simulink model "Task6"  (R2023b)
settings: Solver=FixedStepAuto  StartTime=0.0  StopTime=150  FixedStep=.02  RelTol=1e-3
InitFcn:
  | run("Linear_Model.m")
undefined symbols (not defined in the file or in its folder): A_Lat, A_Long, B_Lat, B_Long, C_Lat, C_Long, D_Lat, D_Long, gravity, sigbuilder_block, states_0, theta0, u0, w0
libraries: simulink_extras x42, cstblocks x27, slpidlib x8
(part 2 of 2)

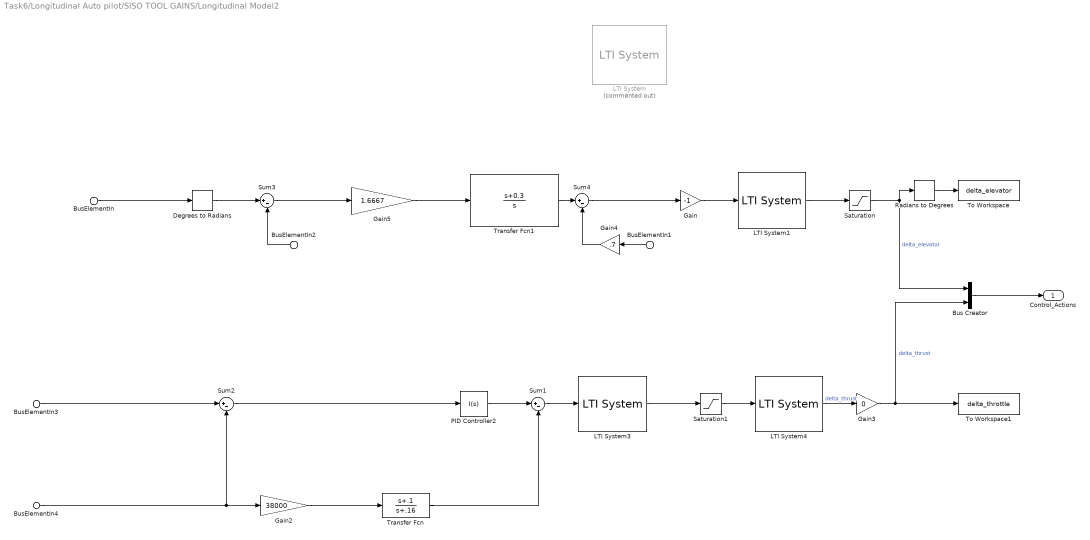
== system Task6/Longitudinal Auto pilot/SISO TOOL GAINS/Longitudinal Model2 ==
  BusElementIn1 : Inport  PortName=deltas  Element=deltas.delta_q
  BusElementIn2 : Inport  PortName=deltas  Element=deltas.delta_theta
  BusElementIn4 : Inport  PortName=deltas  Element=deltas.delta_u
  BusElementIn : Inport  Port=2  PortName=Commands  Element=commands.theta_command
  BusElementIn3 : Inport  Port=2  PortName=Commands  Element=commands.u_command
  Bus Creator : BusCreator  Inputs=2
  Degrees to Radians : simulink_extras/Transformations/Degrees to Radians
  Gain : Gain  Gain=-1
  Gain2 : Gain  Gain=38000
  Gain3 : Gain  Gain=0
  Gain4 : Gain  Gain=.7
  Gain5 : Gain  Gain=1.6667
  LTI System : cstblocks/LTI System  Commented=on  sys=PI_Pitch  IC=[]  PadeOrder=0
  LTI System1 : cstblocks/LTI System  sys=servo  IC=[]  PadeOrder=0
  LTI System3 : cstblocks/LTI System  sys=servo  IC=[]  PadeOrder=0
  LTI System4 : cstblocks/LTI System  sys=Engine_Lag  IC=[]  PadeOrder=0
  PID Controller2 : slpidlib/PID Controller  Controller=I  Form=Parallel  TimeDomain=Continuous-time  UseExternalTs=off  SampleTime=-1  IntegratorMethod=Forward Euler  FilterMethod=Forward Euler  ControllerParametersSource=internal  P=25000  I=1400  UseKiTs=off  D=45918.9077381397  N=24.6739321802593  UseFilter=on  TunerSelectOption=Transfer Function Based (PID Tuner App)  InitialConditionSource=internal  InitialConditionForIntegrator=0  InitialConditionForFilter=0  DifferentiatorICPrevScaledInput=0  ExternalReset=none  TrackingMode=off  Kt=1  LimitOutput=off  SatLimitsSource=internal  UpperSaturationLimit=inf  LowerSaturationLimit=-inf  LinearizeAsGain=on  AntiWindupMode=none  Kb=1  LimitIntegrator=off  UpperIntegratorSaturationLimit=inf  LowerIntegratorSaturationLimit=-inf  POutMin=[]  POutMax=[]  IOutMin=[]  IOutMax=[]  DOutMin=[]  DOutMax=[]  NOutMin=[]  NOutMax=[]  SumOutMin=[]  SumOutMax=[]  SaturationOutMin=[]  SaturationOutMax=[]  PParamMin=[]  PParamMax=[]  IParamMin=[]  IParamMax=[]  DParamMin=[]  DParamMax=[]  NParamMin=[]  NParamMax=[]  KbParamMin=[]  KbParamMax=[]  KtParamMin=[]  KtParamMax=[]  KbOutMin=[]  KbOutMax=[]  KtOutMin=[]  KtOutMax=[]  IntegratorOutMin=[]  IntegratorOutMax=[]  FilterOutMin=[]  FilterOutMax=[]  SumI1OutMin=[]  SumI1OutMax=[]  SumI2OutMin=[]  SumI2OutMax=[]  SumI3OutMin=[]  SumI3OutMax=[]  SumI4OutMin=[]  SumI4OutMax=[]  SumDOutMin=[]  SumDOutMax=[]  DifferentiatorOutMin=[]  DifferentiatorOutMax=[]  FilterDiffOutCoefMin=[]  FilterDiffOutCoefMax=[]  ReciprocalOutMin=[]  ReciprocalOutMax=[]  SumDenOutMin=[]  SumDenOutMax=[]  SumNumOutMin=[]  SumNumOutMax=[]  DivideOutMin=[]  DivideOutMax=[]  UdiffTsProdOutMin=[]  UdiffTsProdOutMax=[]  NTsProdOutMin=[]  NTsProdOutMax=[]  UintegralTsProdOutMin=[]  UintegralTsProdOutMax=[]  UngainTsProdOutMin=[]  UngainTsProdOutMax=[]  ClampingZeroOutDataTypeStr=Inherit: Inherit via back propagation  ClampingZeroOutMin=[]  ClampingZeroOutMax=[]  FilterDenConstantOutDataTypeStr=Inherit: Inherit via back propagation  FilterDenConstantOutMin=[]  FilterDenConstantOutMax=[]  PCopyOutDataTypeStr=Inherit: Inherit via back propagation  PCopyOutMin=[]  PCopyOutMax=[]  NCopyOutDataTypeStr=Inherit: Inherit via back propagation  NCopyOutMin=[]  NCopyOutMax=[]  IntegratorContinuousStateAttributes=''  IntegratorStateMustResolveToSignalObject=off  IntegratorRTWStateStorageClass=Auto  FilterContinuousStateAttributes=''  FilterStateMustResolveToSignalObject=off  FilterRTWStateStorageClass=Auto  ParallelPVariant=Disabled  IdealPVariant=Disabled  IVariant=InternalParameters  DVariant=Disabled  IntegratorVariant=Continuous  SatVariant=Disabled  AWVariant=Passthrough  PCopyVariant=Disabled  TRVariant=Disabled  FdbkBlocksVariant=Forward  IdealPFdbkVariant=Disabled  SatFdbkVariant=Disabled  DerivativeFilterVariant=Disabled  NVariant=Disabled  NCopyVariant=Disabled_SignalSpec  FilterICVariant=Disabled  IntegratorICVariant=InternalICs  ExternalResetVariant=Disabled  TRSumVariant=Passthrough  SumFdbkVariant=Disabled  SumVariant=Passthrough_I  TsampFilterVariant=InternalTs  TsampNgainVariant=Passthrough  TsampIntegralVariant=Disabled_SignalSpec  ExternalSaturationOutDataTypeStr=Inherit: Same as second input
  Radians to Degrees : simulink_extras/Transformations/Radians to Degrees
  Saturation : Saturate  UpperLimit=deg2rad(25)  LowerLimit=deg2rad(-25)
  Saturation1 : Saturate  UpperLimit=65369  LowerLimit=-269369.84
  Sum{1..4} (4 alike) : Sum  Inputs=|+-
  To Workspace : ToWorkspace  VariableName=delta_elevator  SampleTime=-1
  To Workspace1 : ToWorkspace  VariableName=delta_throttle  SampleTime=-1
  Transfer Fcn : TransferFcn  Numerator=[1 .1]  Denominator=[1 .16]
  Transfer Fcn1 : TransferFcn  Numerator=[1 0.3]  Denominator=[1 0]
  Control_Actions : Outport
  wires:
  BusElementIn/1 -> Degrees to Radians/1
  Degrees to Radians/1 -> Sum3/1
  Sum3/1 -> Gain5/1
  Gain/1 -> LTI System1/1
  LTI System1/1 -> Saturation/1
  Saturation/1 -> Bus Creator/1, Radians to Degrees/1  "delta_elevator"
  Bus Creator/1 -> Control_Actions/1
  Radians to Degrees/1 -> To Workspace/1
  Sum2/1 -> PID Controller2/1
  Sum1/1 -> LTI System3/1
  LTI System3/1 -> Saturation1/1
  Saturation1/1 -> LTI System4/1
  Transfer Fcn/1 -> Sum1/2
  LTI System4/1 -> Gain3/1  "delta_thrust"
  Gain2/1 -> Transfer Fcn/1
  PID Controller2/1 -> Sum1/1
  Gain3/1 -> Bus Creator/2, To Workspace1/1  "delta_thrust"
  BusElementIn2/1 -> Sum3/2
  BusElementIn1/1 -> Gain4/1
  BusElementIn3/1 -> Sum2/1
  BusElementIn4/1 -> Sum2/2, Gain2/1
  Gain4/1 -> Sum4/2
  Gain5/1 -> Transfer Fcn1/1
  Sum4/1 -> Gain/1
  Transfer Fcn1/1 -> Sum4/1

== system Task6/Longitudinal Auto pilot/SISO TOOL GAINS/State Space Model3 ==
  Control_Actions : Inport
  Bus Creator1 : BusCreator  Inputs=4
  Bus Selector : BusSelector  OutputSignals=delta_elevator,delta_thrust
  Demux : Demux
  Gain : Gain  Gain=0
  Manual Switch : ManualSwitch
  Mux : Mux  Inputs=2
  State-Space : StateSpace  A=A_Long  B=B_Long  C=C_Long  D=D_Long  InitialCondition=0
  Out Bus Element : Outport  PortName=deltas  Element=deltas
  wires:
  Demux/3 -> Bus Creator1/3  "delta_q"
  Mux/1 -> State-Space/1
  Demux/2 -> Bus Creator1/2  "delta_w"
  Demux/1 -> Bus Creator1/1  "delta_u"
  Bus Creator1/1 -> Out Bus Element/1
  State-Space/1 -> Demux/1
  Demux/4 -> Bus Creator1/4  "delta_theta"
  Manual Switch/1 -> Mux/2
  Gain/1 -> Manual Switch/2
  Control_Actions/1 -> Bus Selector/1
  Bus Selector/1 -> Mux/1  "<delta_elevator>"
  Bus Selector/2 -> Gain/1, Manual Switch/1  "<delta_thrust>"

== system Task6/Longitudinal Auto pilot/SISO TOOL GAINS/Subsystem ==
  Bus Creator2 : BusCreator  Inputs=2
  Constant4 : Constant  Value=15
  Constant5 : Constant  Value=10
  Out Bus Element : Outport  PortName=Commands  Element=commands
  wires:
  Constant4/1 -> Bus Creator2/1  "theta_command"
  Constant5/1 -> Bus Creator2/2  "u_command"
  Bus Creator2/1 -> Out Bus Element/1

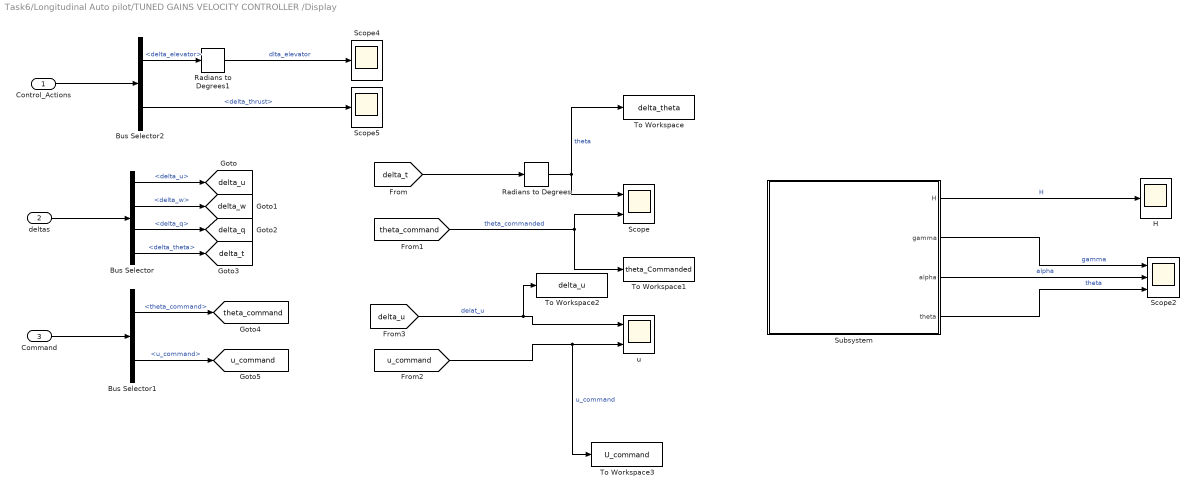
== system Task6/Longitudinal Auto pilot/TUNED GAINS VELOCITY CONTROLLER /Display ==
  Control_Actions : Inport
  deltas : Inport  Port=2
  Command : Inport  Port=3
  Bus Selector : BusSelector  OutputSignals=delta_u,delta_w,delta_q,delta_theta
  Bus Selector1 : BusSelector  OutputSignals=theta_command,u_command
  Bus Selector2 : BusSelector  OutputSignals=delta_elevator,delta_thrust
  H : Scope
  Radians to Degrees : simulink_extras/Transformations/Radians to Degrees
  Radians to Degrees1 : simulink_extras/Transformations/Radians to Degrees
  Scope : Scope  NumInputPorts=2
  Scope2 : Scope  NumInputPorts=3
  Scope4 : Scope
  Scope5 : Scope
  Subsystem : Subsystem
  To Workspace : ToWorkspace  VariableName=delta_theta  SampleTime=-1
  To Workspace1 : ToWorkspace  VariableName=theta_Commanded  SampleTime=-1
  To Workspace2 : ToWorkspace  VariableName=delta_u  SampleTime=-1
  To Workspace3 : ToWorkspace  VariableName=U_command  SampleTime=-1
  u : Scope  NumInputPorts=2
  tag scope: delta_q=global, delta_t=global, delta_u=global, delta_w=global, theta_command=global, u_command=global
  wires:
  deltas/1 -> Bus Selector/1
  Bus Selector/1 -> [delta_u]  "<delta_u>"
  Bus Selector/2 -> [delta_w]  "<delta_w>"
  Bus Selector/3 -> [delta_q]  "<delta_q>"
  Bus Selector/4 -> [delta_t]  "<delta_theta>"
  [delta_t] -> Radians to Degrees/1
  Radians to Degrees/1 -> To Workspace/1, Scope/1  "theta"
  [theta_command] -> To Workspace1/1, Scope/2  "theta_commanded"
  Subsystem/1(H) -> H/1  "H"
  Subsystem/3(alpha) -> Scope2/2  "alpha"
  Subsystem/2(gamma) -> Scope2/1  "gamma"
  Subsystem/4(theta) -> Scope2/3  "theta"
  Command/1 -> Bus Selector1/1
  Bus Selector1/1 -> [theta_command]  "<theta_command>"
  Bus Selector1/2 -> [u_command]  "<u_command>"
  [u_command] -> To Workspace3/1, u/2  "u_command"
  [delta_u] -> To Workspace2/1, u/1  "delat_u"
  Control_Actions/1 -> Bus Selector2/1
  Bus Selector2/1 -> Radians to Degrees1/1  "<delta_elevator>"
  Bus Selector2/2 -> Scope5/1  "<delta_thrust>"
  Radians to Degrees1/1 -> Scope4/1  "dlta_elevator"

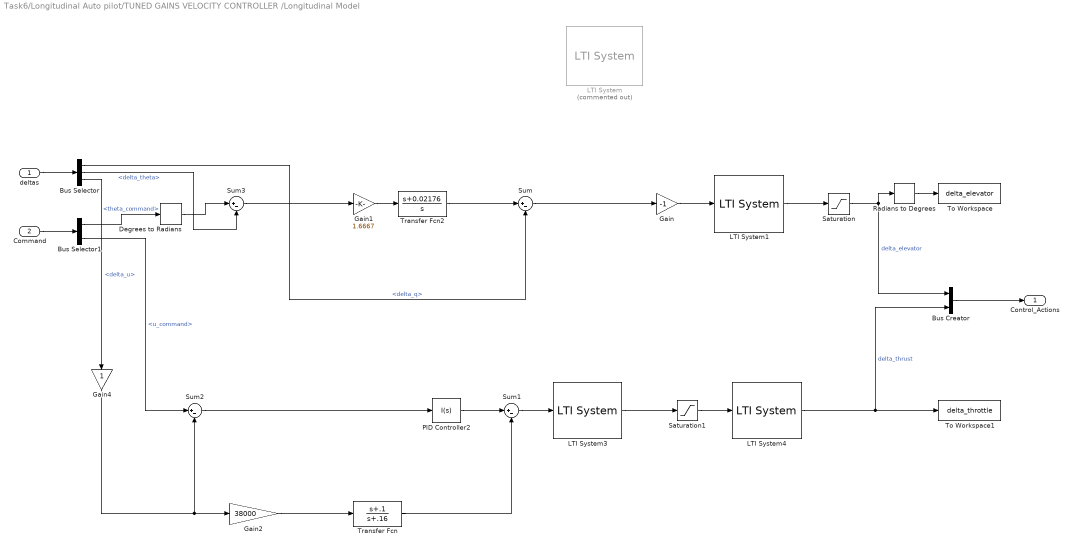
== system Task6/Longitudinal Auto pilot/TUNED GAINS VELOCITY CONTROLLER /Longitudinal Model ==
  deltas : Inport
  Command : Inport  Port=2
  Bus Creator : BusCreator  Inputs=2
  Bus Selector : BusSelector  OutputSignals=delta_q,delta_theta,delta_u
  Bus Selector1 : BusSelector  OutputSignals=theta_command,u_command
  Degrees to Radians : simulink_extras/Transformations/Degrees to Radians
  Gain : Gain  Gain=-1
  Gain1 : Gain  Gain=1.6667
  Gain2 : Gain  Gain=38000
  Gain4 : Gain
  LTI System : cstblocks/LTI System  Commented=on  sys=PI_Pitch  IC=[]  PadeOrder=0
  LTI System1 : cstblocks/LTI System  sys=servo  IC=[]  PadeOrder=0
  LTI System3 : cstblocks/LTI System  sys=servo  IC=[]  PadeOrder=0
  LTI System4 : cstblocks/LTI System  sys=Engine_Lag  IC=[]  PadeOrder=0
  PID Controller2 : slpidlib/PID Controller  Controller=I  Form=Parallel  TimeDomain=Continuous-time  UseExternalTs=off  SampleTime=-1  IntegratorMethod=Forward Euler  FilterMethod=Forward Euler  ControllerParametersSource=internal  P=25000  I=1400  UseKiTs=off  D=45918.9077381397  N=24.6739321802593  UseFilter=on  TunerSelectOption=Transfer Function Based (PID Tuner App)  InitialConditionSource=internal  InitialConditionForIntegrator=0  InitialConditionForFilter=0  DifferentiatorICPrevScaledInput=0  ExternalReset=none  TrackingMode=off  Kt=1  LimitOutput=off  SatLimitsSource=internal  UpperSaturationLimit=inf  LowerSaturationLimit=-inf  LinearizeAsGain=on  AntiWindupMode=none  Kb=1  LimitIntegrator=off  UpperIntegratorSaturationLimit=inf  LowerIntegratorSaturationLimit=-inf  POutMin=[]  POutMax=[]  IOutMin=[]  IOutMax=[]  DOutMin=[]  DOutMax=[]  NOutMin=[]  NOutMax=[]  SumOutMin=[]  SumOutMax=[]  SaturationOutMin=[]  SaturationOutMax=[]  PParamMin=[]  PParamMax=[]  IParamMin=[]  IParamMax=[]  DParamMin=[]  DParamMax=[]  NParamMin=[]  NParamMax=[]  KbParamMin=[]  KbParamMax=[]  KtParamMin=[]  KtParamMax=[]  KbOutMin=[]  KbOutMax=[]  KtOutMin=[]  KtOutMax=[]  IntegratorOutMin=[]  IntegratorOutMax=[]  FilterOutMin=[]  FilterOutMax=[]  SumI1OutMin=[]  SumI1OutMax=[]  SumI2OutMin=[]  SumI2OutMax=[]  SumI3OutMin=[]  SumI3OutMax=[]  SumI4OutMin=[]  SumI4OutMax=[]  SumDOutMin=[]  SumDOutMax=[]  DifferentiatorOutMin=[]  DifferentiatorOutMax=[]  FilterDiffOutCoefMin=[]  FilterDiffOutCoefMax=[]  ReciprocalOutMin=[]  ReciprocalOutMax=[]  SumDenOutMin=[]  SumDenOutMax=[]  SumNumOutMin=[]  SumNumOutMax=[]  DivideOutMin=[]  DivideOutMax=[]  UdiffTsProdOutMin=[]  UdiffTsProdOutMax=[]  NTsProdOutMin=[]  NTsProdOutMax=[]  UintegralTsProdOutMin=[]  UintegralTsProdOutMax=[]  UngainTsProdOutMin=[]  UngainTsProdOutMax=[]  ClampingZeroOutDataTypeStr=Inherit: Inherit via back propagation  ClampingZeroOutMin=[]  ClampingZeroOutMax=[]  FilterDenConstantOutDataTypeStr=Inherit: Inherit via back propagation  FilterDenConstantOutMin=[]  FilterDenConstantOutMax=[]  PCopyOutDataTypeStr=Inherit: Inherit via back propagation  PCopyOutMin=[]  PCopyOutMax=[]  NCopyOutDataTypeStr=Inherit: Inherit via back propagation  NCopyOutMin=[]  NCopyOutMax=[]  IntegratorContinuousStateAttributes=''  IntegratorStateMustResolveToSignalObject=off  IntegratorRTWStateStorageClass=Auto  FilterContinuousStateAttributes=''  FilterStateMustResolveToSignalObject=off  FilterRTWStateStorageClass=Auto  ParallelPVariant=Disabled  IdealPVariant=Disabled  IVariant=InternalParameters  DVariant=Disabled  IntegratorVariant=Continuous  SatVariant=Disabled  AWVariant=Passthrough  PCopyVariant=Disabled  TRVariant=Disabled  FdbkBlocksVariant=Forward  IdealPFdbkVariant=Disabled  SatFdbkVariant=Disabled  DerivativeFilterVariant=Disabled  NVariant=Disabled  NCopyVariant=Disabled_SignalSpec  FilterICVariant=Disabled  IntegratorICVariant=InternalICs  ExternalResetVariant=Disabled  TRSumVariant=Passthrough  SumFdbkVariant=Disabled  SumVariant=Passthrough_I  TsampFilterVariant=InternalTs  TsampNgainVariant=Passthrough  TsampIntegralVariant=Disabled_SignalSpec  ExternalSaturationOutDataTypeStr=Inherit: Same as second input
  Radians to Degrees : simulink_extras/Transformations/Radians to Degrees
  Saturation : Saturate  UpperLimit=deg2rad(25)  LowerLimit=deg2rad(-25)
  Saturation1 : Saturate  UpperLimit=65369  LowerLimit=-269369.84
  Sum{,1..3} (4 alike) : Sum  Inputs=|+-
  To Workspace : ToWorkspace  VariableName=delta_elevator  SampleTime=-1
  To Workspace1 : ToWorkspace  VariableName=delta_throttle  SampleTime=-1
  Transfer Fcn : TransferFcn  Numerator=[1 .1]  Denominator=[1 .16]
  Transfer Fcn2 : TransferFcn  Numerator=[1 0.02176]  Denominator=[1 0]
  Control_Actions : Outport
  wires:
  deltas/1 -> Bus Selector/1
  Command/1 -> Bus Selector1/1
  Bus Selector1/1 -> Degrees to Radians/1  "<theta_command>"
  Bus Selector/2 -> Sum3/2  "<delta_theta>"
  Degrees to Radians/1 -> Sum3/1
  Sum3/1 -> Gain1/1
  Bus Selector/1 -> Sum/2  "<delta_q>"
  Sum/1 -> Gain/1
  Gain/1 -> LTI System1/1
  LTI System1/1 -> Saturation/1
  Saturation/1 -> Bus Creator/1, Radians to Degrees/1  "delta_elevator"
  Bus Creator/1 -> Control_Actions/1
  Radians to Degrees/1 -> To Workspace/1
  Transfer Fcn2/1 -> Sum/1
  Bus Selector/3 -> Gain4/1  "<delta_u>"
  Sum2/1 -> PID Controller2/1
  Sum1/1 -> LTI System3/1
  LTI System3/1 -> Saturation1/1
  Saturation1/1 -> LTI System4/1
  Transfer Fcn/1 -> Sum1/2
  LTI System4/1 -> Bus Creator/2, To Workspace1/1  "delta_thrust"
  Bus Selector1/2 -> Sum2/1  "<u_command>"
  Gain1/1 -> Transfer Fcn2/1
  Gain4/1 -> Sum2/2, Gain2/1
  Gain2/1 -> Transfer Fcn/1
  PID Controller2/1 -> Sum1/1

== system Task6/Longitudinal Auto pilot/TUNED GAINS VELOCITY CONTROLLER /State Space Model ==
  Control_Actions : Inport
  Bus Creator1 : BusCreator  Inputs=4
  Bus Selector : BusSelector  OutputSignals=delta_elevator,delta_thrust
  Demux : Demux
  Gain : Gain  Gain=0
  Manual Switch : ManualSwitch
  Mux : Mux  Inputs=2
  State-Space : StateSpace  A=A_Long  B=B_Long  C=C_Long  D=D_Long  InitialCondition=0
  deltas : Outport
  wires:
  Demux/3 -> Bus Creator1/3  "delta_q"
  Mux/1 -> State-Space/1
  Demux/2 -> Bus Creator1/2  "delta_w"
  Demux/1 -> Bus Creator1/1  "delta_u"
  Bus Creator1/1 -> deltas/1
  State-Space/1 -> Demux/1
  Demux/4 -> Bus Creator1/4  "delta_theta"
  Manual Switch/1 -> Mux/2
  Gain/1 -> Manual Switch/2
  Control_Actions/1 -> Bus Selector/1
  Bus Selector/1 -> Mux/1  "<delta_elevator>"
  Bus Selector/2 -> Gain/1, Manual Switch/1  "<delta_thrust>"

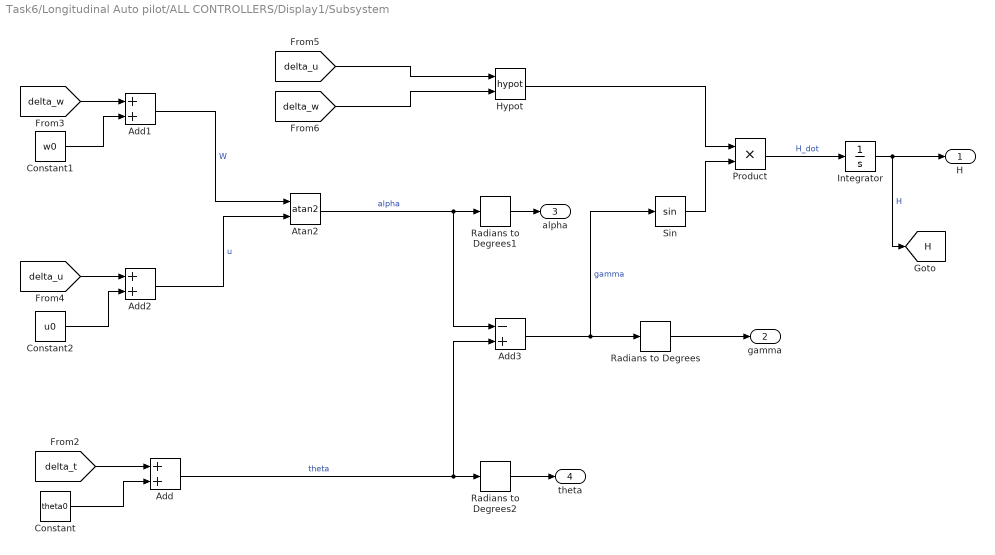
== system Task6/Longitudinal Auto pilot/ALL CONTROLLERS/Display1/Subsystem ==
  Add : Sum
  Add1 : Sum
  Add2 : Sum
  Add3 : Sum  Inputs=-+
  Atan2 : Trigonometry  Operator=atan2
  Constant : Constant  Value=theta0
  Constant1 : Constant  Value=w0
  Constant2 : Constant  Value=u0
  Hypot : Math  Operator=hypot
  Integrator : Integrator  InitialCondition=-states_0(12)
  Product : Product
  Radians to Degrees : simulink_extras/Transformations/Radians to Degrees
  Radians to Degrees1 : simulink_extras/Transformations/Radians to Degrees
  Radians to Degrees2 : simulink_extras/Transformations/Radians to Degrees
  Sin : Trigonometry
  H : Outport
  gamma : Outport  Port=2
  alpha : Outport  Port=3
  theta : Outport  Port=4
  tag scope: H=global
  wires:
  Radians to Degrees2/1 -> theta/1
  Radians to Degrees1/1 -> alpha/1
  Radians to Degrees/1 -> gamma/1
  Add1/1 -> Atan2/1  "W"
  Hypot/1 -> Product/1
  Atan2/1 -> Radians to Degrees1/1, Add3/1  "alpha"
  Add2/1 -> Atan2/2  "u"
  Product/1 -> Integrator/1  "H_dot"
  Add3/1 -> Sin/1, Radians to Degrees/1  "gamma"
  Constant/1 -> Add/2
  Constant2/1 -> Add2/2
  [delta_w] -> Add1/1
  [delta_u] -> Add2/1
  Sin/1 -> Product/2
  Constant1/1 -> Add1/2
  [delta_u] -> Hypot/1
  Add/1 -> Add3/2, Radians to Degrees2/1  "theta"
  [delta_t] -> Add/1
  Integrator/1 -> [H], H/1  "H"
  [delta_w] -> Hypot/2

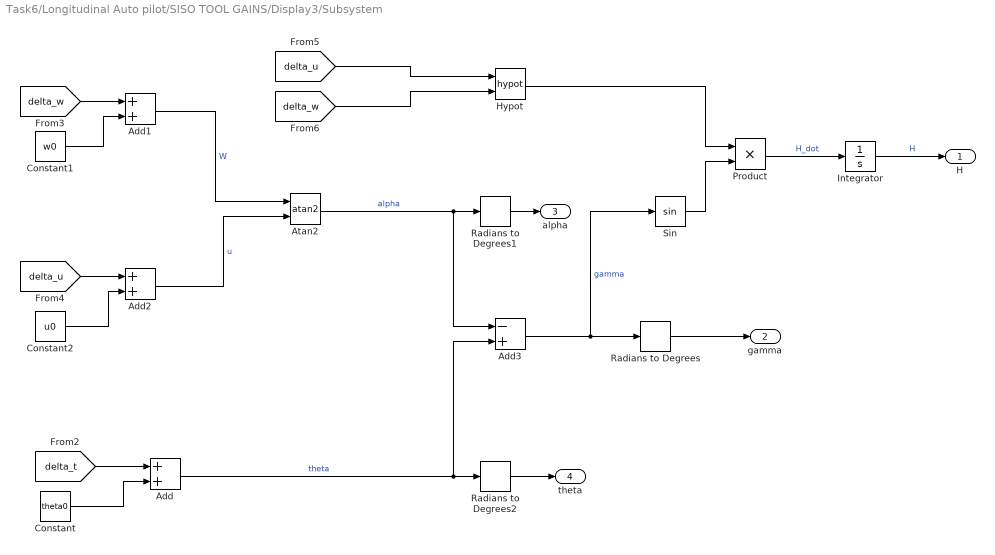
== system Task6/Longitudinal Auto pilot/SISO TOOL GAINS/Display3/Subsystem ==
  Add : Sum
  Add1 : Sum
  Add2 : Sum
  Add3 : Sum  Inputs=-+
  Atan2 : Trigonometry  Operator=atan2
  Constant : Constant  Value=theta0
  Constant1 : Constant  Value=w0
  Constant2 : Constant  Value=u0
  Hypot : Math  Operator=hypot
  Integrator : Integrator  InitialCondition=-states_0(12)
  Product : Product
  Radians to Degrees : simulink_extras/Transformations/Radians to Degrees
  Radians to Degrees1 : simulink_extras/Transformations/Radians to Degrees
  Radians to Degrees2 : simulink_extras/Transformations/Radians to Degrees
  Sin : Trigonometry
  H : Outport
  gamma : Outport  Port=2
  alpha : Outport  Port=3
  theta : Outport  Port=4
  wires:
  [delta_w] -> Hypot/2
  Integrator/1 -> H/1  "H"
  [delta_t] -> Add/1
  Add/1 -> Radians to Degrees2/1, Add3/2  "theta"
  [delta_u] -> Hypot/1
  Constant1/1 -> Add1/2
  Sin/1 -> Product/2
  [delta_u] -> Add2/1
  [delta_w] -> Add1/1
  Constant2/1 -> Add2/2
  Constant/1 -> Add/2
  Add3/1 -> Radians to Degrees/1, Sin/1  "gamma"
  Product/1 -> Integrator/1  "H_dot"
  Add2/1 -> Atan2/2  "u"
  Atan2/1 -> Add3/1, Radians to Degrees1/1  "alpha"
  Hypot/1 -> Product/1
  Add1/1 -> Atan2/1  "W"
  Radians to Degrees/1 -> gamma/1
  Radians to Degrees1/1 -> alpha/1
  Radians to Degrees2/1 -> theta/1

== system Task6/Longitudinal Auto pilot/TUNED GAINS VELOCITY CONTROLLER /Display/Subsystem ==
  Add : Sum
  Add1 : Sum
  Add2 : Sum
  Add3 : Sum  Inputs=-+
  Atan2 : Trigonometry  Operator=atan2
  Constant : Constant  Value=theta0
  Constant1 : Constant  Value=w0
  Constant2 : Constant  Value=u0
  Hypot : Math  Operator=hypot
  Integrator : Integrator  InitialCondition=-states_0(12)
  Product : Product
  Radians to Degrees : simulink_extras/Transformations/Radians to Degrees
  Radians to Degrees1 : simulink_extras/Transformations/Radians to Degrees
  Radians to Degrees2 : simulink_extras/Transformations/Radians to Degrees
  Sin : Trigonometry
  H : Outport
  gamma : Outport  Port=2
  alpha : Outport  Port=3
  theta : Outport  Port=4
  wires:
  [delta_w] -> Hypot/2
  Integrator/1 -> H/1  "H"
  [delta_t] -> Add/1
  Add/1 -> Radians to Degrees2/1, Add3/2  "theta"
  [delta_u] -> Hypot/1
  Constant1/1 -> Add1/2
  Sin/1 -> Product/2
  [delta_u] -> Add2/1
  [delta_w] -> Add1/1
  Constant2/1 -> Add2/2
  Constant/1 -> Add/2
  Add3/1 -> Radians to Degrees/1, Sin/1  "gamma"
  Product/1 -> Integrator/1  "H_dot"
  Add2/1 -> Atan2/2  "u"
  Atan2/1 -> Add3/1, Radians to Degrees1/1  "alpha"
  Hypot/1 -> Product/1
  Add1/1 -> Atan2/1  "W"
  Radians to Degrees/1 -> gamma/1
  Radians to Degrees1/1 -> alpha/1
  Radians to Degrees2/1 -> theta/1
